simulink model "RocketStateSpace"  (R2024b)
settings: Solver=VariableStepAuto  StartTime=0.0  StopTime=25  RelTol=1e-3
model workspace (MAT data in the model file):
  Thrust = 1
values from neighbouring files (symbols this model uses):
  K = lqr(A, B, Q, R)    [State_Control_Matrices.m]
libraries: simulink x5
settings Model: Creator=liesb  LastModifiedBy=liesb

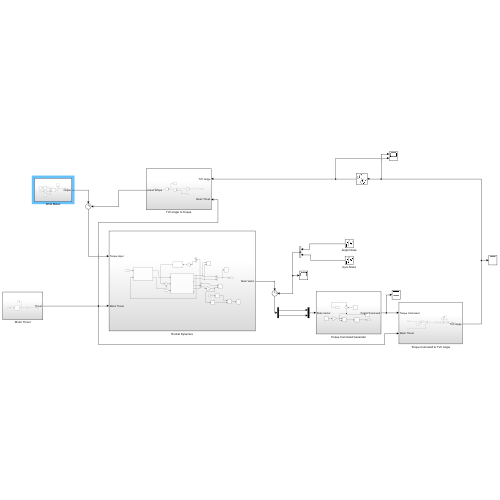
[thumbnail: Simulink's stored preview of the top-level diagram]
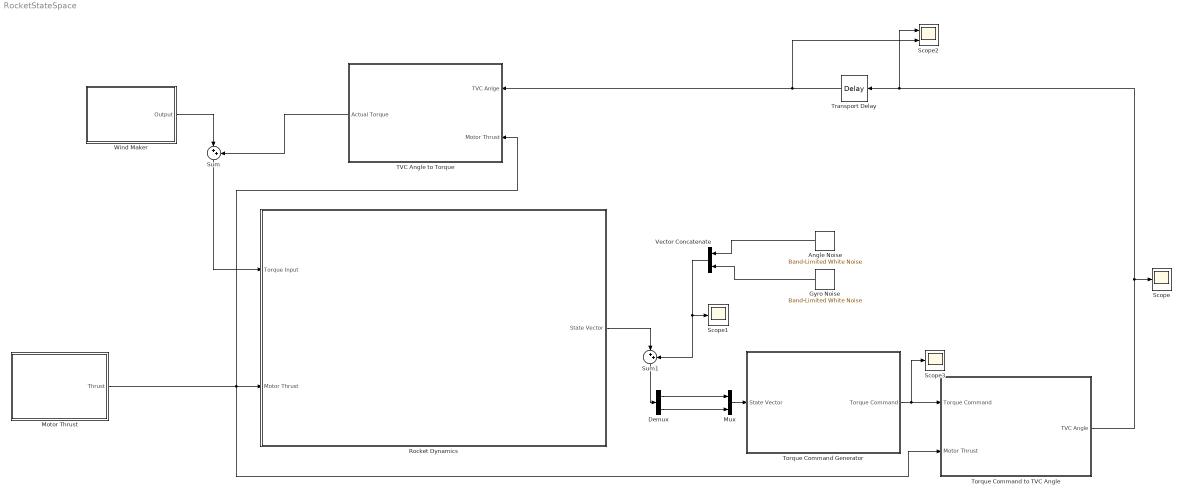
== system RocketStateSpace ==
  Angle Noise : simulink/Sources/Band-Limited White Noise  Cov=[6.9e-8]  Ts=0.01  seed=[23341]
  Demux : Demux  Outputs=2
  Gyro Noise : simulink/Sources/Band-Limited White Noise  Cov=[0]  Ts=0.01  seed=[12345]
  Motor Thrust : Subsystem
  Mux : Mux  Inputs=2
  Rocket Dynamics : Subsystem
  Scope : Scope
  Scope1 : Scope
  Scope2 : Scope  NumInputPorts=2
  Scope3 : Scope
  Sum : Sum  Inputs=|++
  Sum1 : Sum  Inputs=|++
  TVC Angle to Torque : Subsystem
  Torque Command Generator : Subsystem
  Torque Command to TVC Angle : Subsystem
  Transport Delay : TransportDelay  DelayTime=0.09
  Vector Concatenate : Concatenate
  Wind Maker : Subsystem
  wires:
  Motor Thrust/1(Thrust) -> Torque Command to TVC Angle/2(Motor Thrust), TVC Angle to Torque/2(Motor Thrust), Rocket Dynamics/2(Motor Thrust)
  Torque Command Generator/1(Torque Command) -> Scope3/1, Torque Command to TVC Angle/1(Torque Command)
  TVC Angle to Torque/1(Actual Torque) -> Sum/2
  Angle Noise/1 -> Vector Concatenate/1
  Vector Concatenate/1 -> Sum1/2, Scope1/1
  Rocket Dynamics/1(State Vector) -> Sum1/1
  Wind Maker/1(Output) -> Sum/1
  Torque Command to TVC Angle/1(TVC Angle) -> Transport Delay/1, Scope2/1, Scope/1
  Sum/1 -> Rocket Dynamics/1(Torque Input)
  Gyro Noise/1 -> Vector Concatenate/2
  Sum1/1 -> Demux/1
  Demux/1 -> Mux/1
  Demux/2 -> Mux/2
  Mux/1 -> Torque Command Generator/1(State Vector)
  Transport Delay/1 -> Scope2/2, TVC Angle to Torque/1(TVC Anlge)

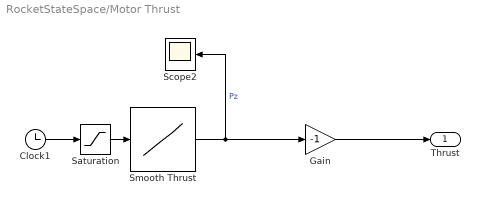
== system RocketStateSpace/Motor Thrust ==
  Clock1 : Clock
  Gain : Gain  Gain=-1
  Saturation : Saturate  UpperLimit=4.35  LowerLimit=0
  Scope2 : Scope
  Smooth Thrust : Lookup_n-D  NumberOfTableDimensions=1  BreakpointsForDimension1=[0;0.050000000000000003;0.10000000000000001;0.20000000000000001;0.5;1;2;3;3.2999999999999998;3.6000000000000001;3.8999999999999999;4.3499999999999996]  Table=[40;62;40;38;40;39;38;37;36;30;15;0]  InterpMethod=Akima spline  InternalRulePriority=Speed  RndMeth=Simplest
  Thrust : Outport
  wires:
  Smooth Thrust/1 -> Gain/1, Scope2/1  "Pz"
  Clock1/1 -> Saturation/1
  Saturation/1 -> Smooth Thrust/1
  Gain/1 -> Thrust/1

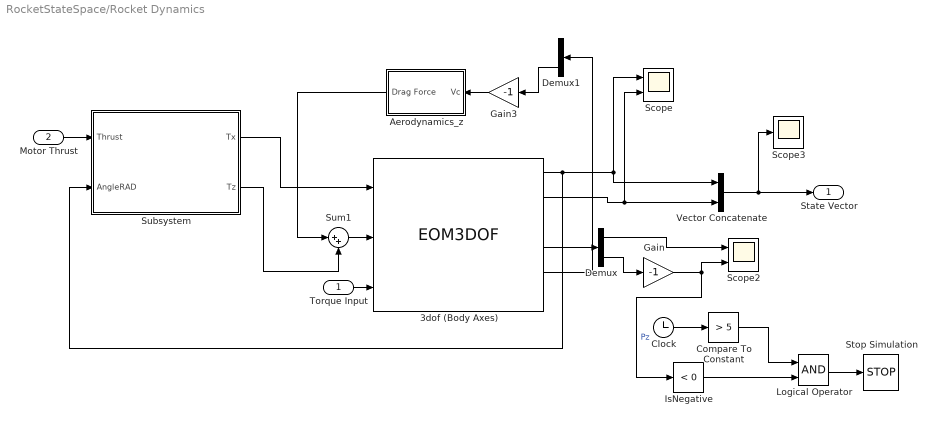
== system RocketStateSpace/Rocket Dynamics ==
  Torque Input : Inport
  Motor Thrust : Inport  Port=2
  3dof (Body Axes) : EOM3DOF  v_ini=0  mass=1.35  Iyy=0.0857
  Aerodynamics_z : Subsystem
  Clock : Clock
  Compare To Constant : simulink/Logic and Bit Operations/Compare To Constant  relop=>  const=5  OutDataTypeStr=boolean
  Demux : Demux  Outputs=2
  Demux1 : Demux  Outputs=2
  Gain : Gain  Gain=-1
  Gain3 : Gain  Gain=-1
  IsNegative : simulink/Logic and Bit Operations/Compare To Zero  relop=<  OutDataTypeStr=boolean
      settings: LibrarySourceBlock=|
      | simulink/Quick Insert/Logic and Bit
      | Operations/IsNegative
  Logical Operator : Logic  AllPortsSameDT=off  OutDataTypeStr=boolean
  Scope : Scope  NumInputPorts=2
  Scope2 : Scope  NumInputPorts=2
  Scope3 : Scope
  Stop Simulation : Stop
  Subsystem : Subsystem
  Sum1 : Sum  Inputs=|++
  Vector Concatenate : Concatenate
  State Vector : Outport
  wires:
  3dof (Body Axes)/2 -> Scope/2, Vector Concatenate/2
  Gain/1 -> IsNegative/1, Scope2/2  "Pz"
  Demux1/2 -> Gain3/1
  Clock/1 -> Compare To Constant/1
  IsNegative/1 -> Logical Operator/2
  Demux/1 -> Scope2/1
  Gain3/1 -> Aerodynamics_z/1(Vc)
  Demux/2 -> Gain/1
  Compare To Constant/1 -> Logical Operator/1
  3dof (Body Axes)/1 -> Subsystem/2(AngleRAD), Scope/1, Vector Concatenate/1
  Subsystem/1(Tx) -> 3dof (Body Axes)/1
  3dof (Body Axes)/5 -> Demux1/1
  Aerodynamics_z/1(Drag Force) -> Sum1/1
  Logical Operator/1 -> Stop Simulation/1
  Sum1/1 -> 3dof (Body Axes)/2
  3dof (Body Axes)/4 -> Demux/1
  Subsystem/2(Tz) -> Sum1/2
  Vector Concatenate/1 -> Scope3/1, State Vector/1
  Torque Input/1 -> 3dof (Body Axes)/3
  Motor Thrust/1 -> Subsystem/1(Thrust)

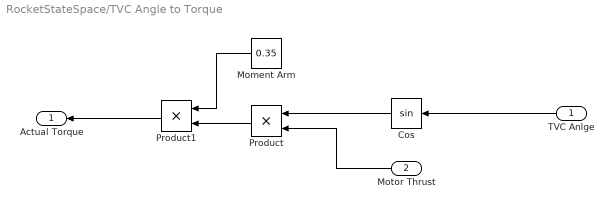
== system RocketStateSpace/TVC Angle to Torque ==
  TVC Anlge : Inport
  Motor Thrust : Inport  Port=2
  Cos : Trigonometry
  Moment Arm : Constant  Value=0.35
  Product : Product
  Product1 : Product
  Actual Torque : Outport
  wires:
  TVC Anlge/1 -> Cos/1
  Product/1 -> Product1/2
  Moment Arm/1 -> Product1/1
  Product1/1 -> Actual Torque/1
  Cos/1 -> Product/1
  Motor Thrust/1 -> Product/2

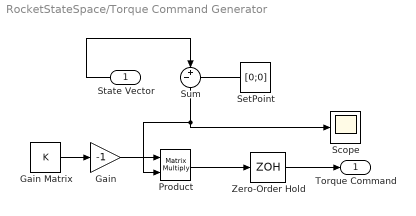
== system RocketStateSpace/Torque Command Generator ==
  State Vector : Inport
  Gain : Gain  Gain=-1
  Gain Matrix : Constant  Value=K  VectorParams1D=off
  Product : Product  Multiplication=Matrix(*)
  Scope : Scope
  SetPoint : Constant  Value=[0;0]
  Sum : Sum  Inputs=|+-
  Zero-Order Hold : ZeroOrderHold  SampleTime=0.01
  Torque Command : Outport
  wires:
  Product/1 -> Zero-Order Hold/1
  SetPoint/1 -> Sum/2
  Sum/1 -> Scope/1, Product/2
  Gain Matrix/1 -> Gain/1
  State Vector/1 -> Sum/1
  Gain/1 -> Product/1
  Zero-Order Hold/1 -> Torque Command/1

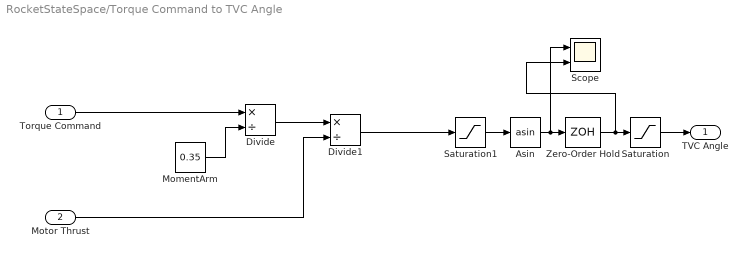
== system RocketStateSpace/Torque Command to TVC Angle ==
  Torque Command : Inport
  Motor Thrust : Inport  Port=2
  Asin : Trigonometry  Operator=asin
  Divide : Product  Inputs=*/
  Divide1 : Product  Inputs=*/
  MomentArm : Constant  Value=0.35
  Saturation : Saturate  UpperLimit=0.087  LowerLimit=-0.087
  Saturation1 : Saturate  UpperLimit=1  LowerLimit=-1
  Scope : Scope  NumInputPorts=2
  Zero-Order Hold : ZeroOrderHold  SampleTime=0.01
  TVC Angle : Outport
  wires:
  Divide1/1 -> Saturation1/1
  Asin/1 -> Scope/1, Zero-Order Hold/1
  Divide/1 -> Divide1/1
  Zero-Order Hold/1 -> Scope/2, Saturation/1
  MomentArm/1 -> Divide/2
  Torque Command/1 -> Divide/1
  Saturation/1 -> TVC Angle/1
  Saturation1/1 -> Asin/1
  Motor Thrust/1 -> Divide1/2

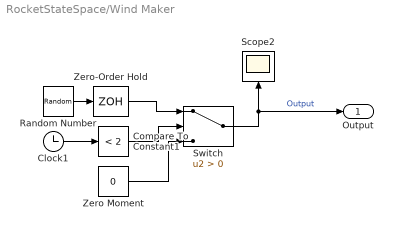
== system RocketStateSpace/Wind Maker ==
  Clock1 : Clock
  Compare To Constant1 : simulink/Logic and Bit Operations/Compare To Constant  relop=<  const=2  OutDataTypeStr=boolean
  Random Number : RandomNumber  Variance=0.04  Seed=420  SampleTime=0.01
  Scope2 : Scope
  Switch : Switch  Criteria=u2 > Threshold  SaturateOnIntegerOverflow=off  InputSameDT=off
  Zero Moment : Constant  Value=0
  Zero-Order Hold : ZeroOrderHold  SampleTime=0.5
  Output : Outport
  wires:
  Random Number/1 -> Zero-Order Hold/1
  Compare To Constant1/1 -> Switch/2
  Switch/1 -> Output/1, Scope2/1  "Output"
  Clock1/1 -> Compare To Constant1/1
  Zero-Order Hold/1 -> Switch/1
  Zero Moment/1 -> Switch/3

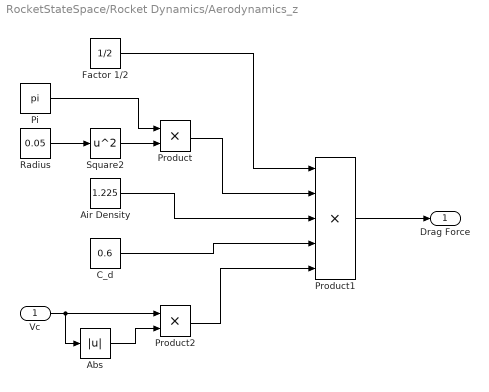
== system RocketStateSpace/Rocket Dynamics/Aerodynamics_z ==
  Vc : Inport
  Abs : Abs  SaturateOnIntegerOverflow=off
  Air Density : Constant  Value=1.225
  C_d : Constant  Value=0.6
  Factor 1/2 : Constant  Value=1/2
  Pi : Constant  Value=pi  OutDataTypeStr=Inherit: Inherit via back propagation
  Product : Product
  Product1 : Product  Inputs=5
  Product2 : Product
  Radius : Constant  Value=0.05
  Square2 : Math  Operator=square  SignedPower=on  RndMeth=Zero
  Drag Force : Outport
  wires:
  Vc/1 -> Product2/1, Abs/1
  Radius/1 -> Square2/1
  Pi/1 -> Product/1
  Square2/1 -> Product/2
  Factor 1/2/1 -> Product1/1
  Product/1 -> Product1/2
  Air Density/1 -> Product1/3
  C_d/1 -> Product1/4
  Product1/1 -> Drag Force/1
  Product2/1 -> Product1/5
  Abs/1 -> Product2/2

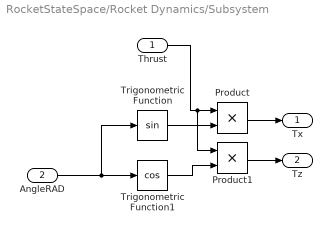
== system RocketStateSpace/Rocket Dynamics/Subsystem ==
  Thrust : Inport
  AngleRAD : Inport  Port=2
  Product : Product
  Product1 : Product
  Trigonometric Function : Trigonometry
  Trigonometric Function1 : Trigonometry  Operator=cos
  Tx : Outport
  Tz : Outport  Port=2
  wires:
  AngleRAD/1 -> Trigonometric Function1/1, Trigonometric Function/1
  Thrust/1 -> Product1/1, Product/1
  Trigonometric Function/1 -> Product/2
  Trigonometric Function1/1 -> Product1/2
  Product1/1 -> Tz/1
  Product/1 -> Tx/1
